simulink model "Calibrating_The_AR_Drone_Sensors_Model"  (R2016a)
settings: Solver=FixedStepDiscrete  StartTime=0.0  StopTime=inf  FixedStep=1/400  RelTol=1e-3
libraries: AR_Drone_Sensors x2
settings Model: DataDictionary=ArDroneDataDictionary.sldd  SimulationMode=external  ExtModeTrigDuration=100000  Creator=sannem  LastModifiedBy=sbyebss
settings ConfigSet: Description=This configuration set can be used to generate code that runs on the Parrot AR Drone 2.0 in External mode.
settings SolverCC: PositivePriorityOrder=on
settings DataIOCC: LimitDataPoints=on  SaveFormat=Array
settings OptimizationCC: OptimizeModelRefInitCode=on  LifeSpan=1  MaxStackSize=64
settings DebuggingCC: UnderspecifiedInitializationDetection=Classic  MergeDetectMultiDrivingBlocksExec=none  InheritedTsInSrcMsg=none  ParameterPrecisionLossMsg=none
settings HardwareCC: ProdBitPerPointer=32  ProdLargestAtomicInteger=Long  ProdLargestAtomicFloat=Double  ProdIntDivRoundTo=Undefined  ProdWordSize=32  ProdHWDeviceType=ARM Compatible->ARM Cortex
settings ModelReferenceCC: PropagateSignalLabelsOutOfModel=off
settings SFSimCC: SimCustomHeaderCode="#include \"IMU_Navdata.h\""
settings RTWCC: SystemTargetFile=ert.tlc  HardwareBoard=AR Drone 2 - Thread Timer Scheduler  TemplateMakefile=ert_default_tmf  Toolchain=Code Sourcery
settings CodeAppCC: IgnoreCustomStorageClasses=off  MaxIdLength=63
settings ERTTargetCC: SupportComplex=off  ExtMode=on  ExtModeMexArgs=extModeParams  ConvertIfToSwitch=off  SuppressUnreachableDefaultCases=off
settings ConfigComp: CovModelRefEnable=Off  CovSFcnEnable=off

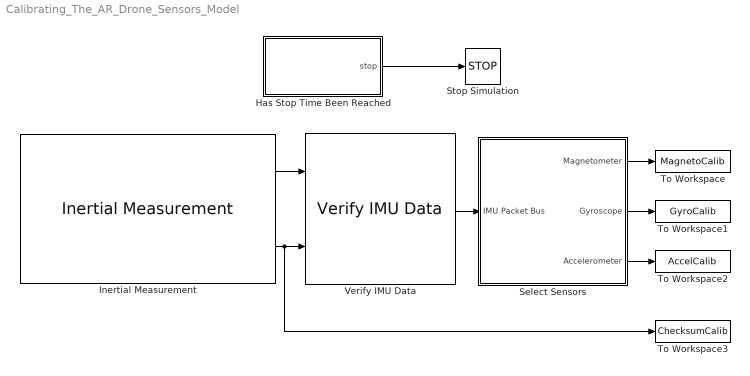
== system Calibrating_The_AR_Drone_Sensors_Model ==
  Has Stop Time Been Reached : MATLAB Function  TreatAsAtomicUnit=on  SystemSampleTime=sampleTime  mask{stopTime=60, sampleTime=1/200}
      mask prompts: stopTime "Stop time [s]"; sampleTime "Sample time [s]"
      mask help: This block will keep track of the run time of a model. The default output is "0" with the output changing to "1" if the run time exceeds the user specified stop time.
  Inertial Measurement : AR_Drone_Sensors/Inertial Measurement  Ts=1/200
  Select Sensors : Subsystem
  Stop Simulation : Stop
  To Workspace : ToWorkspace  VariableName=MagnetoCalib  SaveFormat=Structure With Time  SampleTime=-1
  To Workspace1 : ToWorkspace  VariableName=GyroCalib  SaveFormat=Structure With Time  SampleTime=-1
  To Workspace2 : ToWorkspace  VariableName=AccelCalib  SaveFormat=Structure With Time  SampleTime=-1
  To Workspace3 : ToWorkspace  VariableName=ChecksumCalib  SaveFormat=Structure With Time  SampleTime=-1
  Verify IMU Data : AR_Drone_Sensors/Verify IMU Data
  wires:
  Has Stop Time Been Reached/1(stop) -> Stop Simulation/1
  Verify IMU Data/1 -> Select Sensors/1(IMU Packet Bus)
  Select Sensors/1(Magnetometer) -> To Workspace/1
  Select Sensors/2(Gyroscope) -> To Workspace1/1
  Select Sensors/3(Accelerometer) -> To Workspace2/1
  Inertial Measurement/2 -> Verify IMU Data/2, To Workspace3/1
  Inertial Measurement/1 -> Verify IMU Data/1

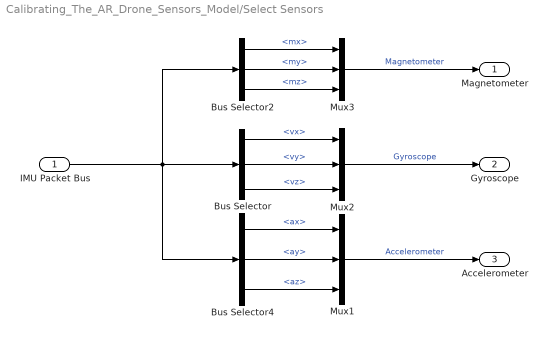
== system Calibrating_The_AR_Drone_Sensors_Model/Select Sensors ==
  IMU Packet Bus : Inport  OutDataTypeStr=Bus: IMU_Packets
  Bus Selector : BusSelector  OutputSignals=vx,vy,vz
  Bus Selector2 : BusSelector  OutputSignals=mx,my,mz
  Bus Selector4 : BusSelector  OutputSignals=ax,ay,az
  Mux1 : Mux  Inputs=3
  Mux2 : Mux  Inputs=3
  Mux3 : Mux  Inputs=3
  Magnetometer : Outport
  Gyroscope : Outport  Port=2
  Accelerometer : Outport  Port=3
  wires:
  Bus Selector/3 -> Mux2/3  "<vz>"
  Bus Selector/2 -> Mux2/2  "<vy>"
  Bus Selector/1 -> Mux2/1  "<vx>"
  Bus Selector2/3 -> Mux3/3  "<mz>"
  Bus Selector2/2 -> Mux3/2  "<my>"
  Bus Selector2/1 -> Mux3/1  "<mx>"
  Bus Selector4/3 -> Mux1/3  "<az>"
  Bus Selector4/2 -> Mux1/2  "<ay>"
  Bus Selector4/1 -> Mux1/1  "<ax>"
  IMU Packet Bus/1 -> Bus Selector4/1, Bus Selector/1, Bus Selector2/1
  Mux1/1 -> Accelerometer/1  "Accelerometer"
  Mux2/1 -> Gyroscope/1  "Gyroscope"
  Mux3/1 -> Magnetometer/1  "Magnetometer"

== matlab function Calibrating_The_AR_Drone_Sensors_Model/Has Stop Time Been Reached ==
  data: stop output; stopTime parameter; sampleTime parameter
function stop = stopTimeReached(stopTime,sampleTime)
%#codegen

% persistent variable which keeps track of the total run time
persistent runTime
if isempty(runTime)
    runTime = sampleTime
else
    runTime = runTime + sampleTime;
end

stop = 0;
% verify whether the stop time is reached
if runTime > stopTime
    stop = 1;
end
